simulink model "niof_model"  (R2021a)
settings: Solver=ode23tb  StartTime=0.0  StopTime=2  RelTol=1e-3
values from neighbouring files (symbols this model uses):
  h0 = ds.DateTime(1).Hour + ds.DateTime(1).Minute/60    [compiler_niof_model.m]
  S_area_hole = 0.01    [set_params_blocks.m]
undefined symbols (not defined in the file or in its folder): crop_GH1_NFT_slot1___C, crop_GH1_NFT_slot1___N, crop_GH1_NFT_slot1___R, crop_GH1_NFT_slot2___C, crop_GH1_NFT_slot2___N, crop_GH1_NFT_slot2___R, crop_GH1_NFT_slot3___C, crop_GH1_NFT_slot3___N, crop_GH1_NFT_slot3___R, crop_GH1_NFT_slot4___C, crop_GH1_NFT_slot4___N, crop_GH1_NFT_slot4___R, crop_GH1_RF_slot1___C, crop_GH1_RF_slot1___N, crop_GH1_RF_slot1___R, crop_GH1_RF_slot2___C, crop_GH1_RF_slot2___N, crop_GH1_RF_slot2___R, crop_GH1_RF_slot3___C, crop_GH1_RF_slot3___N, crop_GH1_RF_slot3___R, crop_GH1_RF_slot4___C, crop_GH1_RF_slot4___N, crop_GH1_RF_slot4___R, crop_GH2_RF_slot1___C, crop_GH2_RF_slot1___N, crop_GH2_RF_slot1___R, crop_GH2_RF_slot2___C, crop_GH2_RF_slot2___N, crop_GH2_RF_slot2___R, crop_GH2_RF_slot3___C, crop_GH2_RF_slot3___N, crop_GH2_RF_slot3___R, crop_GH2_RF_slot4___C, crop_GH2_RF_slot4___N, crop_GH2_RF_slot4___R, crop_GH2_TRAD_slot1___C, crop_GH2_TRAD_slot1___N, crop_GH2_TRAD_slot1___R, crop_GH2_TRAD_slot2___C, crop_GH2_TRAD_slot2___N, crop_GH2_TRAD_slot2___R, crop_GH2_TRAD_slot3___C, crop_GH2_TRAD_slot3___N, crop_GH2_TRAD_slot3___R, crop_GH2_TRAD_slot4___C, crop_GH2_TRAD_slot4___N, crop_GH2_TRAD_slot4___R, fish, GH3_Tank1_tend, GH3_Tank2_tend, GH3_Tank3_tend, GH3_Tank4_tend, tp_biofilter___T, tp_fish_C___T, tp_fish_M___T, tp_fish_S___T, tp_fish_T___T, tp_GH1_bio___T, tp_GH1_NFT___T ... (+3)
libraries: HORTISIM x152
(part 1 of 4)
settings Model: Creator=djoroya  LastModifiedBy=djoroya
settings SolverCC: MinimalZcImpactIntegration=on
settings DataIOCC: SaveFormat=StructureWithTime  ReturnWorkspaceOutputsName=tpa3f80949_6031_4c8f_ac4c_761b248f1577
settings DebuggingCC: UnconnectedInputMsg=none  UnconnectedOutputMsg=none  UnconnectedLineMsg=none  UnderSpecifiedDimensionMsg=warning
settings HardwareCC: TargetBitPerLong=64  TargetBitPerPointer=64  TargetBitPerSizeT=64  TargetBitPerPtrDiffT=64  TargetLongLongMode=on  TargetIntDivRoundTo=Zero  TargetEndianess=LittleEndian  TargetWordSize=64  TargetHWDeviceType=MATLAB Host  ProdEqTarget=off
settings RTWCC: Description=Rapid Simulation Target  SystemTargetFile=rsim.tlc  TemplateMakefile=rsim_default_tmf
settings CodeAppCC: GenerateComments=off  SimulinkBlockComments=off
settings RSimTargetCC: TargetLangStandard=C99 (ISO)

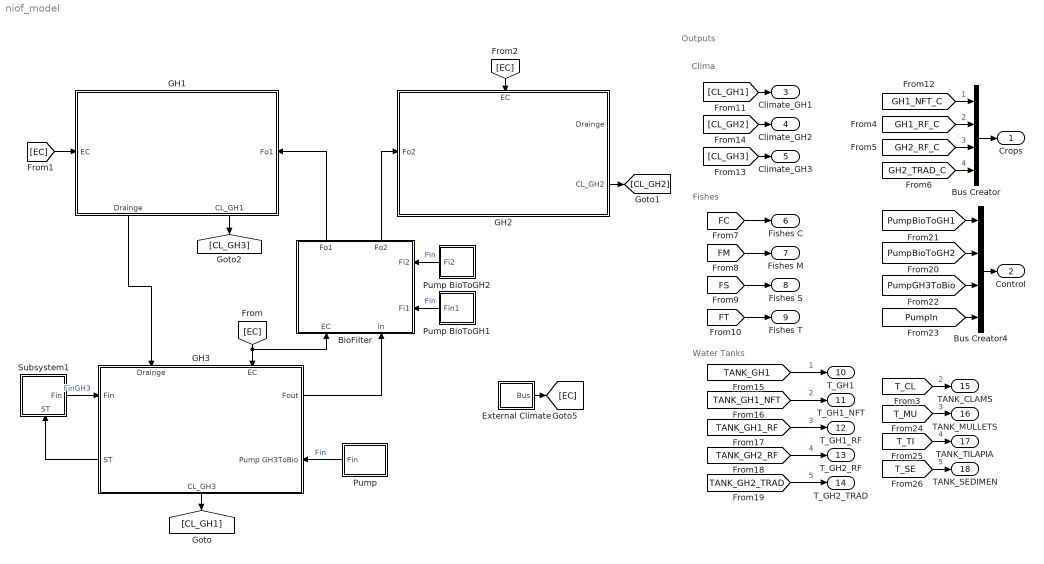
== system niof_model ==
  note: Clima
  note: Water Tanks
  note: Outputs
  note: Fishes
  BioFilter : Subsystem
      settings: PortSchema="{\"entries\":[{\"content\":{\"sides\":[{\"content\":{\"connectorIds\":[]},\"type\":\"ConnectorPlacement.EquallySpacedRectSide\",\"uuid\":\"39de7e6f-241b-402f-a120-18892c124752\"},{\"content\":{\"connectorIds\":[\"In3\",\"In4\"],\"side\":\"RIGHT\"},\"type\":\"ConnectorPlacement.EquallySpacedRectSide\",\"uuid\":\"cefc2988-7ee7-4e24-926e-b8e4989b17f9\"},{\"content\":{\"connectorIds\":[\"Out1\",\"Out2\"],\"side\":\"TOP\"},\"type\":\"ConnectorPlacement.EquallySpacedRectSide\",\"uuid\":\"4036c4c8-5802-453b-98d5-164c4771b92f\"},{\"content\":{\"connectorIds\":[\"In1\",\"In2\"],\"side\":\"BOTTOM\"},\"type\":\"ConnectorPlacement.EquallySpacedRectSide\",\"uuid\":\"379a93f8-bf00-465a-a0f2-a3fe498cb65a\"}]},\"type\":\"ConnectorPlacement.EquallySpacedConnector\",\"uuid\":\"a3e40081-564f-4c6d-9212-7fcf3036ef72\"}],\"packageUris\":[\"http://schema.mathworks.com/mf0/Connector/R2020b\"],\"version\":\"1.0\"}"
  Bus Creator : BusCreator  Inputs=4
  Bus Creator4 : BusCreator  Inputs=4
  External Climate : Subsystem
  GH1 : Subsystem
      settings: PortSchema="{\"entries\":[{\"content\":{\"sides\":[{\"content\":{\"connectorIds\":[\"In1\"]},\"type\":\"ConnectorPlacement.EquallySpacedRectSide\",\"uuid\":\"f96e7fae-faa6-4c45-94ca-623160b74f18\"},{\"content\":{\"connectorIds\":[\"In2\"],\"side\":\"RIGHT\"},\"type\":\"ConnectorPlacement.EquallySpacedRectSide\",\"uuid\":\"cb53bd10-123e-4148-bfa4-80436b7b153d\"},{\"content\":{\"connectorIds\":[],\"side\":\"TOP\"},\"type\":\"ConnectorPlacement.EquallySpacedRectSide\",\"uuid\":\"63bb56bc-b382-4b43-9081-bb2d51c32075\"},{\"content\":{\"connectorIds\":[\"Out1\",\"Out2\"],\"side\":\"BOTTOM\"},\"type\":\"ConnectorPlacement.EquallySpacedRectSide\",\"uuid\":\"67dc5313-4d07-4554-a853-f934e5f830b0\"}]},\"type\":\"ConnectorPlacement.EquallySpacedConnector\",\"uuid\":\"a823a839-de0c-41cf-8d5c-d5714b085e52\"}],\"packageUris\":[\"http://schema.mathworks.com/mf0/Connector/R2020b\"],\"version\":\"1.0\"}"
  GH2 : Subsystem
      settings: PortSchema="{\"entries\":[{\"content\":{\"sides\":[{\"content\":{\"connectorIds\":[\"In1\"]},\"type\":\"ConnectorPlacement.EquallySpacedRectSide\",\"uuid\":\"f96e7fae-faa6-4c45-94ca-623160b74f18\"},{\"content\":{\"connectorIds\":[\"Out1\",\"Out2\"],\"side\":\"RIGHT\"},\"type\":\"ConnectorPlacement.EquallySpacedRectSide\",\"uuid\":\"cb53bd10-123e-4148-bfa4-80436b7b153d\"},{\"content\":{\"connectorIds\":[\"In2\"],\"side\":\"TOP\"},\"type\":\"ConnectorPlacement.EquallySpacedRectSide\",\"uuid\":\"63bb56bc-b382-4b43-9081-bb2d51c32075\"},{\"content\":{\"connectorIds\":[],\"side\":\"BOTTOM\"},\"type\":\"ConnectorPlacement.EquallySpacedRectSide\",\"uuid\":\"67dc5313-4d07-4554-a853-f934e5f830b0\"}]},\"type\":\"ConnectorPlacement.EquallySpacedConnector\",\"uuid\":\"a823a839-de0c-41cf-8d5c-d5714b085e52\"}],\"packageUris\":[\"http://schema.mathworks.com/mf0/Connector/R2020b\"],\"version\":\"1.0\"}"
  GH3 : Subsystem
      settings: PortSchema="{\"entries\":[{\"content\":{\"sides\":[{\"content\":{\"connectorIds\":[\"In1\",\"Out3\"]},\"type\":\"ConnectorPlacement.EquallySpacedRectSide\",\"uuid\":\"81ee264a-41e1-40c0-ab1d-9f5a989c7824\"},{\"content\":{\"connectorIds\":[\"Out1\",\"In4\"],\"side\":\"RIGHT\"},\"type\":\"ConnectorPlacement.EquallySpacedRectSide\",\"uuid\":\"6f93fb8e-2d1c-4265-8b9a-fc3ac97daf53\"},{\"content\":{\"connectorIds\":[\"In2\",\"In3\"],\"side\":\"TOP\"},\"type\":\"ConnectorPlacement.EquallySpacedRectSide\",\"uuid\":\"a3cd6f92-7543-4360-a672-0bbe0cd8561c\"},{\"content\":{\"connectorIds\":[\"Out2\"],\"side\":\"BOTTOM\"},\"type\":\"ConnectorPlacement.EquallySpacedRectSide\",\"uuid\":\"24dd70c2-9a78-443d-9f3d-70d95e180355\"}]},\"type\":\"ConnectorPlacement.EquallySpacedConnector\",\"uuid\":\"c2201d0a-197a-46d7-9039-6a7936abb698\"}],\"packageUris\":[\"http://schema.mathworks.com/mf0/Connector/R2020b\"],\"version\":\"1.0\"}"
  Pump : Subsystem
  Pump BioToGH1 : Subsystem
  Pump BioToGH2 : Subsystem
  Subsystem1 : Subsystem
      settings: PortSchema="{\"entries\":[{\"content\":{\"sides\":[{\"content\":{\"connectorIds\":[]},\"type\":\"ConnectorPlacement.EquallySpacedRectSide\",\"uuid\":\"9a0d525f-008d-4bea-82c7-ff44bdf3c7a1\"},{\"content\":{\"connectorIds\":[\"Out1\"],\"side\":\"RIGHT\"},\"type\":\"ConnectorPlacement.EquallySpacedRectSide\",\"uuid\":\"3b01d65a-c3f3-4d47-b396-44b5c3b80049\"},{\"content\":{\"connectorIds\":[],\"side\":\"TOP\"},\"type\":\"ConnectorPlacement.EquallySpacedRectSide\",\"uuid\":\"5f7d9f63-0ae7-4a14-b423-83c3827e552d\"},{\"content\":{\"connectorIds\":[\"In1\"],\"side\":\"BOTTOM\"},\"type\":\"ConnectorPlacement.EquallySpacedRectSide\",\"uuid\":\"b4e81995-be21-4f86-9bdb-ec727bfc31aa\"}]},\"type\":\"ConnectorPlacement.EquallySpacedConnector\",\"uuid\":\"2d17a637-3468-41a4-99e0-95edda826c96\"}],\"packageUris\":[\"http://schema.mathworks.com/mf0/Connector/R2020b\"],\"version\":\"1.0\"}"
  Crops : Outport  PortDimensions=62*4*4
  Control : Outport  Port=2
  Climate_GH1 : Outport  Port=3
  Climate_GH2 : Outport  Port=4
  Climate_GH3 : Outport  Port=5
  Fishes C : Outport  Port=6
  Fishes M : Outport  Port=7
  Fishes S : Outport  Port=8
  Fishes T : Outport  Port=9
  T_GH1 : Outport  Port=10
  T_GH1_NFT : Outport  Port=11
  T_GH1_RF : Outport  Port=12
  T_GH2_RF : Outport  Port=13
  T_GH2_TRAD : Outport  Port=14
  TANK_CLAMS : Outport  Port=15
  TANK_MULLETS : Outport  Port=16
  TANK_TILAPIA : Outport  Port=17
  TANK_SEDIMEN : Outport  Port=18
  wires:
  Subsystem1/1(Fin) -> GH3/1(Fin)  "FinGH3"
  Pump/1(Fin) -> GH3/4(Pump GH3ToBio)  "Fin"
  External Climate/1(Bus) -> [EC]
  [EC] -> BioFilter/1(EC), GH3/3(EC)
  Pump BioToGH1/1(Fin1) -> BioFilter/4(Fi1)  "Fin"
  Pump BioToGH2/1(Fi2) -> BioFilter/3(Fi2)  "Fin"
  GH3/1(Fout) -> BioFilter/2(in)
  [EC] -> GH1/1(EC)
  [EC] -> GH2/2(EC)
  BioFilter/1(Fo1) -> GH1/2(Fo1)
  BioFilter/2(Fo2) -> GH2/1(Fo2)
  GH1/1(Drainge) -> GH3/2(Drainge)
  GH3/3(ST) -> Subsystem1/1(ST)
  Bus Creator/1 -> Crops/1
  [GH1_NFT_C] -> Bus Creator/1  "1"
  [GH1_RF_C] -> Bus Creator/2  "2"
  [GH2_RF_C] -> Bus Creator/3  "3"
  [GH2_TRAD_C] -> Bus Creator/4  "4"
  [FC] -> Fishes C/1
  [FM] -> Fishes M/1
  [FS] -> Fishes S/1
  [FT] -> Fishes T/1
  [TANK_GH1_NFT] -> T_GH1_NFT/1  "2"
  [TANK_GH1_RF] -> T_GH1_RF/1  "3"
  [TANK_GH2_RF] -> T_GH2_RF/1  "4"
  [TANK_GH2_TRAD] -> T_GH2_TRAD/1  "5"
  [PumpBioToGH1] -> Bus Creator4/1
  [PumpBioToGH2] -> Bus Creator4/2
  [PumpGH3ToBio] -> Bus Creator4/3
  [PumpIn] -> Bus Creator4/4
  Bus Creator4/1 -> Control/1
  [TANK_GH1] -> T_GH1/1  "1"
  GH3/2(CL_GH3) -> [CL_GH1]
  GH2/2(CL_GH2) -> [CL_GH2]
  GH1/2(CL_GH1) -> [CL_GH3]
  [CL_GH1] -> Climate_GH1/1
  [CL_GH2] -> Climate_GH2/1
  [CL_GH3] -> Climate_GH3/1
  [T_CL] -> TANK_CLAMS/1  "2"
  [T_MU] -> TANK_MULLETS/1  "3"
  [T_SE] -> TANK_SEDIMEN/1  "5"
  [T_TI] -> TANK_TILAPIA/1  "4"

== system niof_model/BioFilter ==
  EC : Inport
  in : Inport  Port=2
  Fi2 : Inport  Port=3
  Fi1 : Inport  Port=4
  Bio Filter : Subsystem
  Bus Selector : BusSelector  OutputSignals=Fout
  Parse : Subsystem
  Selector : Selector  InputPortWidth=2  IndexOptions=Index vector (dialog)  Indices=[1]  OutputSizes=1
  Selector1 : Selector  InputPortWidth=2  IndexOptions=Index vector (dialog)  Indices=[2]  OutputSizes=1
  Tank Model Bio : HORTISIM/Aquaculture/Models/Tank Model  S=tp_biofilter___S  h_max=tp_biofilter___h_max  wall_gain=tp_biofilter___wall_gain  ThermalConductivityWall=tp_biofilter___ThermalConductivityWall  Tsubwall=tp_biofilter___Tsubwall  h=tp_biofilter___h  X=tp_biofilter___X  T=tp_biofilter___T  Twall=tp_biofilter___Twall  d_t=tp_biofilter___d_t
      settings: SourceProductName=Horti Simulator
      mask Display: image('water_tank.png'); % Use "Edit Image" on toolstrip to change.
  Vector Concatenate : Concatenate  Mode=Multidimensional array
  Zero Element Flow : HORTISIM/Other  Functions/Zero Element Flow  SystemSampleTime=-1  VariantActivationTime=update diagram  Latency=0  AutoFrameSizeCalculation=off
      settings: SourceProductName=Horti Simulator
  Fo1 : Outport
  Fo2 : Outport  Port=2
  wires:
  Fi2/1 -> Vector Concatenate/2
  in/1 -> Tank Model Bio/1
  Parse/1(Clima) -> Tank Model Bio/3
  Bus Selector/1 -> Selector/1, Selector1/1  "<Fout>"
  Zero Element Flow/1 -> Tank Model Bio/2
  Selector1/1 -> Fo2/1
  Tank Model Bio/1 -> Bus Selector/1  "WT Bio"
  EC/1 -> Parse/1(EC)
  Vector Concatenate/1 -> Tank Model Bio/4
  Fi1/1 -> Vector Concatenate/1
  Selector/1 -> Fo1/1
  Bio Filter/1(Out1) -> Tank Model Bio/5

== system niof_model/External Climate ==
  Constant : Constant  Value=440
  Demux : Demux
  From Workspace : FromWorkspace  VariableName=S01_EC
  Scalar2Bus ExternalClimate : HORTISIM/Other  Functions/Scalar2Bus ExternalClimate  SystemSampleTime=-1  VariantActivationTime=update diagram  Latency=0  AutoFrameSizeCalculation=off
      settings: SourceProductName=Horti Simulator
  Bus : Outport
  wires:
  Scalar2Bus ExternalClimate/1 -> Bus/1
  Demux/3 -> Scalar2Bus ExternalClimate/3
  Demux/1 -> Scalar2Bus ExternalClimate/1
  Demux/2 -> Scalar2Bus ExternalClimate/2
  Constant/1 -> Scalar2Bus ExternalClimate/5
  Demux/4 -> Scalar2Bus ExternalClimate/4
  From Workspace/1 -> Demux/1

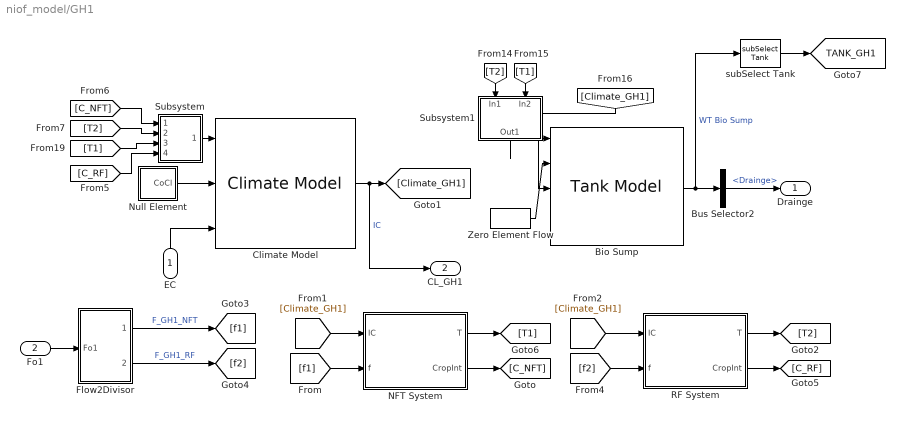
== system niof_model/GH1 ==
  EC : Inport
  Fo1 : Inport  Port=2
  Bio Sump : HORTISIM/Aquaculture/Models/Tank Model  S=tp_GH1_bio___S  h_max=tp_GH1_bio___h_max  wall_gain=tp_GH1_bio___wall_gain  ThermalConductivityWall=tp_GH1_bio___ThermalConductivityWall  Tsubwall=tp_GH1_bio___Tsubwall  h=tp_GH1_bio___h  X=tp_GH1_bio___X  T=tp_GH1_bio___T  Twall=tp_GH1_bio___Twall  d_t=tp_GH1_bio___d_t
      settings: SourceProductName=Horti Simulator
  Bus Selector2 : BusSelector  OutputSignals=Drainge
  Climate Model : HORTISIM/Climate/Models/Climate Model  hour0=climate_GH1___hour0  G0=climate_GH1___G0  T0=climate_GH1___T0  H=climate_GH1___H  A_f=climate_GH1___A_f  A_c=climate_GH1___A_c  minWindows=climate_GH1___minWindows  lam_s=climate_GH1___lam_s  c_s=climate_GH1___c_s  l_s=climate_GH1___l_s  rhod_s=climate_GH1___rhod_s  int_air_speed=climate_GH1___int_air_speed  alpha_i=climate_GH1___alpha_i  alpha_c=climate_GH1___alpha_c  tau_c=climate_GH1___tau_c  alpha_f=climate_GH1___alpha_f  d_c=climate_GH1___d_c  cd_c=climate_GH1___cd_c  T_ss=climate_GH1___T_ss
      settings: SourceProductName=Horti Simulator
  Flow2Divisor : Subsystem
  NFT System : Subsystem
  Null Element : Subsystem
  RF System : Subsystem
  Subsystem : Subsystem
  Subsystem1 : Subsystem
  Zero Element Flow : HORTISIM/Other  Functions/Zero Element Flow  SystemSampleTime=-1  VariantActivationTime=update diagram  Latency=0  AutoFrameSizeCalculation=off
      settings: SourceProductName=Horti Simulator
  subSelect Tank : HORTISIM/Other  Functions/subSelect  Tank  SystemSampleTime=-1  VariantActivationTime=update diagram  Latency=0  AutoFrameSizeCalculation=off
      settings: SourceProductName=Horti Simulator
  Drainge : Outport
  CL_GH1 : Outport  Port=2
  tag scope: TANK_GH1=global
  wires:
  Fo1/1 -> Flow2Divisor/1(Fo1)
  Flow2Divisor/1(Out1) -> [f1]  "F_GH1_NFT"
  Flow2Divisor/2(Out2) -> [f2]  "F_GH1_RF"
  [f2] -> RF System/2(f)
  [Climate_GH1] -> RF System/1(IC)
  RF System/1(T) -> [T2]
  [f1] -> NFT System/2(f)
  [Climate_GH1] -> NFT System/1(IC)
  NFT System/1(T) -> [T1]
  RF System/2(CropInt) -> [C_RF]
  NFT System/2(CropInt) -> [C_NFT]
  Null Element/1(CoCl) -> Climate Model/2
  Climate Model/1 -> CL_GH1/1, [Climate_GH1]  "IC"
  EC/1 -> Climate Model/3
  [C_NFT] -> Subsystem/1(In1)
  [T2] -> Subsystem/2(In2)
  [T1] -> Subsystem/3(In3)
  [C_RF] -> Subsystem/4(In4)
  Subsystem/1(CoCl) -> Climate Model/1
  Zero Element Flow/1 -> Bio Sump/2
  Bus Selector2/1 -> Drainge/1  "<Drainge>"
  Bio Sump/1 -> subSelect Tank/1, Bus Selector2/1  "WT Bio Sump"
  [Climate_GH1] -> Bio Sump/3
  [T2] -> Subsystem1/1(In1)
  [T1] -> Subsystem1/2(In2)
  Subsystem1/1(Out1) -> Bio Sump/1
  subSelect Tank/1 -> [TANK_GH1]

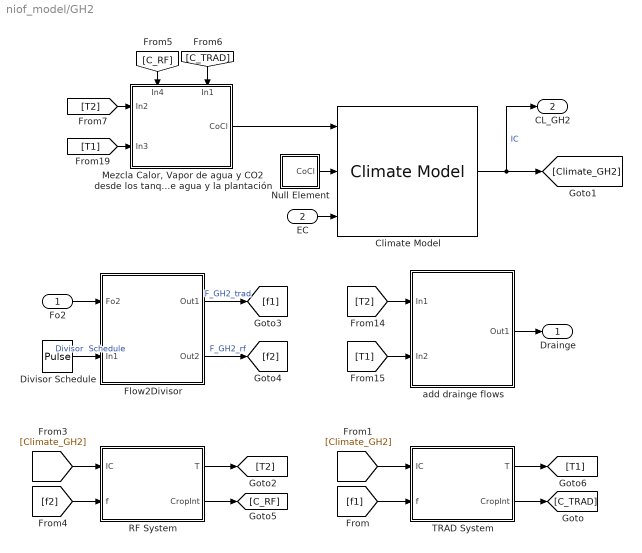
== system niof_model/GH2 ==
  Fo2 : Inport
  EC : Inport  Port=2
  Climate Model : HORTISIM/Climate/Models/Climate Model  hour0=climate_GH2___hour0  G0=climate_GH2___G0  T0=climate_GH2___T0  H=climate_GH2___H  A_f=climate_GH2___A_f  A_c=climate_GH2___A_c  minWindows=climate_GH2___minWindows  lam_s=climate_GH2___lam_s  c_s=climate_GH2___c_s  l_s=climate_GH2___l_s  rhod_s=climate_GH2___rhod_s  int_air_speed=climate_GH2___int_air_speed  alpha_i=climate_GH2___alpha_i  alpha_c=climate_GH2___alpha_c  tau_c=climate_GH2___tau_c  alpha_f=climate_GH2___alpha_f  d_c=climate_GH2___d_c  cd_c=climate_GH2___cd_c  T_ss=climate_GH2___T_ss
      settings: SourceProductName=Horti Simulator
  Divisor Schedule : DiscretePulseGenerator  PulseType=Time based  Period=7  PulseWidth=100/7  PhaseDelay=8/24-h0
  Flow2Divisor : Subsystem
  "Mezcla Calor, Vapor de agua y CO2 desde los tanques de agua y la plantación" : Subsystem
      settings: PortSchema="{\"entries\":[{\"content\":{\"sides\":[{\"content\":{\"connectorIds\":[\"In1\",\"In2\"]},\"type\":\"ConnectorPlacement.EquallySpacedRectSide\",\"uuid\":\"19434035-201c-4d1e-b085-add0f5d76683\"},{\"content\":{\"connectorIds\":[\"Out1\"],\"side\":\"RIGHT\"},\"type\":\"ConnectorPlacement.EquallySpacedRectSide\",\"uuid\":\"bba1eca2-c9f3-4d99-84f3-6a563e445b18\"},{\"content\":{\"connectorIds\":[\"In3\",\"In4\"],\"side\":\"TOP\"},\"type\":\"ConnectorPlacement.EquallySpacedRectSide\",\"uuid\":\"0c3973cd-a057-4788-9737-1d39699ad24a\"}]},\"type\":\"ConnectorPlacement.EquallySpacedConnector\",\"uuid\":\"7a49bd96-3016-4969-a817-6dbc9b87987e\"}],\"packageUris\":[\"http://schema.mathworks.com/mf0/Connector/R2020b\"],\"version\":\"1.0\"}"
  Null Element : Subsystem
  RF System : Subsystem
  TRAD System : Subsystem
  add drainge flows : Subsystem
  Drainge : Outport
  CL_GH2 : Outport  Port=2
  wires:
  Fo2/1 -> Flow2Divisor/1(Fo2)
  Flow2Divisor/1(Out1) -> [f1]  "F_GH2_trad"
  Flow2Divisor/2(Out2) -> [f2]  "F_GH2_rf"
  Divisor Schedule/1 -> Flow2Divisor/2(In1)  "Divisor  Schedule"
  [f2] -> RF System/2(f)
  [Climate_GH2] -> TRAD System/1(IC)
  RF System/1(T) -> [T2]
  [Climate_GH2] -> RF System/1(IC)
  RF System/2(CropInt) -> [C_RF]
  TRAD System/2(CropInt) -> [C_TRAD]
  TRAD System/1(T) -> [T1]
  [f1] -> TRAD System/2(f)
  Null Element/1(CoCl) -> Climate Model/2
  Climate Model/1 -> CL_GH2/1, [Climate_GH2]  "IC"
  EC/1 -> Climate Model/3
  [C_TRAD] -> "Mezcla Calor, Vapor de agua y CO2 desde los tanques de agua y la plantación"/4(In1)
  [T2] -> "Mezcla Calor, Vapor de agua y CO2 desde los tanques de agua y la plantación"/1(In2)
  [T1] -> "Mezcla Calor, Vapor de agua y CO2 desde los tanques de agua y la plantación"/2(In3)
  [C_RF] -> "Mezcla Calor, Vapor de agua y CO2 desde los tanques de agua y la plantación"/3(In4)
  "Mezcla Calor, Vapor de agua y CO2 desde los tanques de agua y la plantación"/1(CoCl) -> Climate Model/1
  [T2] -> add drainge flows/1(In1)
  [T1] -> add drainge flows/2(In2)
  add drainge flows/1(Out1) -> Drainge/1

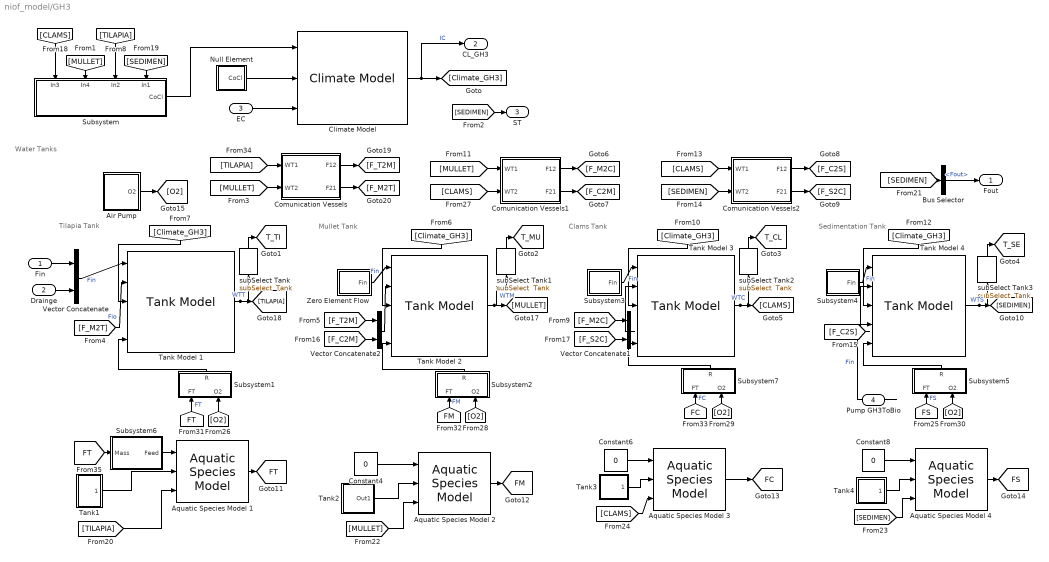
== system niof_model/GH3 ==
  note: Water Tanks
  note: Tilapia Tank
  note: Clams Tank
  note: Mullet Tank
  note: Sedimentation Tank
  Fin : Inport
  Drainge : Inport  Port=2
  EC : Inport  Port=3
  Pump GH3ToBio : Inport  Port=4
  Air Pump : Subsystem
  Aquatic Species Model 1 : HORTISIM/Aquaculture/Models/Aquatic Species Model  rfish=ratio.tilapia  mfishsat=mass_sat.tilapia  a_max=GH3_Tank1_tend + 1  a0=0  m0=fish.tilapia.Mass(1)  A_R=1e-3*[1 0 0 0 0 0 -1 1]'  B_R=1e-3*[1 0 0 0 0 0 -1 1]'
      settings: SourceProductName=Horti Simulator
  Aquatic Species Model 2 : HORTISIM/Aquaculture/Models/Aquatic Species Model  rfish=ratio.mullet  mfishsat=mass_sat.mullet  a_max=GH3_Tank2_tend + 1  a0=0  m0=fish.mullet.Mass(1)  A_R=1e-3*[1 0 0 0 0 0 -1 1]'  B_R=1e-3*[1 0 0 0 0 0 -1 1]'
      settings: SourceProductName=Horti Simulator
  Aquatic Species Model 3 : HORTISIM/Aquaculture/Models/Aquatic Species Model  rfish=ratio.clams  mfishsat=mass_sat.clams  a_max=GH3_Tank3_tend + 1  a0=0  m0=fish.clams.Mass(1)  A_R=1e-3*[1 0 0 0 0 0 -1 1]'  B_R=1e-3*[1 0 0 0 0 0 -1 1]'
      settings: SourceProductName=Horti Simulator
  Aquatic Species Model 4 : HORTISIM/Aquaculture/Models/Aquatic Species Model  rfish=ratio.silver  mfishsat=mass_sat.silver  a_max=GH3_Tank4_tend + 1  a0=0  m0=fish.silver.Mass(1)  A_R=1e-3*[1 0 0 0 0 0 -1 1]'  B_R=1e-3*[1 0 0 0 0 0 -1 1]'
      settings: SourceProductName=Horti Simulator
  Bus Selector : BusSelector  OutputSignals=Fout
  Climate Model : HORTISIM/Climate/Models/Climate Model  hour0=climate_GH3___hour0  G0=climate_GH3___G0  T0=climate_GH3___T0  H=climate_GH3___H  A_f=climate_GH3___A_f  A_c=climate_GH3___A_c  minWindows=climate_GH3___minWindows  lam_s=climate_GH3___lam_s  c_s=climate_GH3___c_s  l_s=climate_GH3___l_s  rhod_s=climate_GH3___rhod_s  int_air_speed=climate_GH3___int_air_speed  alpha_i=climate_GH3___alpha_i  alpha_c=climate_GH3___alpha_c  tau_c=climate_GH3___tau_c  alpha_f=climate_GH3___alpha_f  d_c=climate_GH3___d_c  cd_c=climate_GH3___cd_c  T_ss=climate_GH3___T_ss
      settings: SourceProductName=Horti Simulator
  Comunication Vessels : Subsystem  mask{S=S_area_hole}
  Comunication Vessels1 : Subsystem  mask{S=S_area_hole}
  Comunication Vessels2 : Subsystem  mask{S=S_area_hole}
  Constant4 : Constant  Value=0
  Constant6 : Constant  Value=0
  Constant8 : Constant  Value=0
  Null Element : Subsystem
  Subsystem : Subsystem
      settings: PortSchema="{\"entries\":[{\"content\":{\"sides\":[{\"content\":{\"connectorIds\":[]},\"type\":\"ConnectorPlacement.EquallySpacedRectSide\",\"uuid\":\"d0110122-4c0e-4050-9905-351100dfb2f8\"},{\"content\":{\"connectorIds\":[\"Out1\"],\"side\":\"RIGHT\"},\"type\":\"ConnectorPlacement.EquallySpacedRectSide\",\"uuid\":\"5eb4c138-aba2-4968-a926-5140e929ef74\"},{\"content\":{\"connectorIds\":[\"In1\",\"In2\",\"In3\",\"In4\"],\"side\":\"TOP\"},\"type\":\"ConnectorPlacement.EquallySpacedRectSide\",\"uuid\":\"102db217-6442-4bf3-9377-05d6ceeffd2a\"}]},\"type\":\"ConnectorPlacement.EquallySpacedConnector\",\"uuid\":\"fec43415-4143-4543-8db6-6efa996130a9\"}],\"packageUris\":[\"http://schema.mathworks.com/mf0/Connector/R2020b\"],\"version\":\"1.0\"}"
  Subsystem1 : Subsystem
  Subsystem2 : Subsystem
  Subsystem3 : Subsystem
  Subsystem4 : Subsystem
  Subsystem5 : Subsystem
  Subsystem6 : Subsystem  mask{FCR=1e-4}
  Subsystem7 : Subsystem
  Tank Model 1 : HORTISIM/Aquaculture/Models/Tank Model  S=tp_fish_T___S  h_max=tp_fish_T___h_max  wall_gain=tp_fish_T___wall_gain  ThermalConductivityWall=tp_fish_T___ThermalConductivityWall  Tsubwall=tp_fish_T___Tsubwall  h=tp_fish_T___h  X=tp_fish_T___X  T=tp_fish_T___T  Twall=tp_fish_T___Twall  d_t=tp_fish_T___d_t
      settings: SourceProductName=Horti Simulator
  Tank Model 2 : HORTISIM/Aquaculture/Models/Tank Model  S=tp_fish_M___S  h_max=tp_fish_M___h_max  wall_gain=tp_fish_M___wall_gain  ThermalConductivityWall=tp_fish_M___ThermalConductivityWall  Tsubwall=tp_fish_M___Tsubwall  h=tp_fish_M___h  X=tp_fish_M___X  T=tp_fish_M___T  Twall=tp_fish_M___Twall  d_t=tp_fish_M___d_t
      settings: SourceProductName=Horti Simulator
      mask Display: image('water_tank.png'); % Use "Edit Image" on toolstrip to change.
  Tank Model 3 : HORTISIM/Aquaculture/Models/Tank Model  S=tp_fish_C___S  h_max=tp_fish_C___h_max  wall_gain=tp_fish_C___wall_gain  ThermalConductivityWall=tp_fish_C___ThermalConductivityWall  Tsubwall=tp_fish_C___Tsubwall  h=tp_fish_C___h  X=tp_fish_C___X  T=tp_fish_C___T  Twall=tp_fish_C___Twall  d_t=tp_fish_C___d_t
      settings: SourceProductName=Horti Simulator
      mask Display: image('water_tank.png'); % Use "Edit Image" on toolstrip to change.
  Tank Model 4 : HORTISIM/Aquaculture/Models/Tank Model  S=tp_fish_S___S  h_max=tp_fish_S___h_max  wall_gain=tp_fish_S___wall_gain  ThermalConductivityWall=tp_fish_S___ThermalConductivityWall  Tsubwall=tp_fish_S___Tsubwall  h=tp_fish_S___h  X=tp_fish_S___X  T=tp_fish_S___T  Twall=tp_fish_S___Twall  d_t=tp_fish_S___d_t
      settings: SourceProductName=Horti Simulator
      mask Display: image('water_tank.png'); % Use "Edit Image" on toolstrip to change.
  Tank1 : Subsystem
  Tank2 : Subsystem
  Tank3 : Subsystem
  Tank4 : Subsystem
  Vector Concatenate : Concatenate  Mode=Multidimensional array
  Vector Concatenate1 : Concatenate
  Vector Concatenate2 : Concatenate
  Zero Element Flow : Subsystem
  subSelect Tank{,1..3} (4 alike) : HORTISIM/Other  Functions/subSelect  Tank  SystemSampleTime=-1  VariantActivationTime=update diagram  Latency=0  AutoFrameSizeCalculation=off
      settings: SourceProductName=Horti Simulator
  Fout : Outport
  CL_GH3 : Outport  Port=2
  ST : Outport  Port=3
  tag scope: FC=global, FM=global, FS=global, FT=global, T_CL=global, T_MU=global, T_SE=global, T_TI=global
  wires:
  EC/1 -> Climate Model/3
  [SEDIMEN] -> Subsystem/4(In1)
  Climate Model/1 -> CL_GH3/1, [Climate_GH3]  "IC"
  Subsystem/1(CoCl) -> Climate Model/1
  [CLAMS] -> Subsystem/1(In3)
  [MULLET] -> Subsystem/2(In4)
  [TILAPIA] -> Subsystem/3(In2)
  Null Element/1(CoCl) -> Climate Model/2
  Fin/1 -> Vector Concatenate/1
  Drainge/1 -> Vector Concatenate/2
  [SEDIMEN] -> ST/1
  Bus Selector/1 -> Fout/1  "<Fout>"
  Subsystem5/1(R) -> Tank Model 4/5
  [FS] -> Subsystem5/1(FT)  "FS"
  [O2] -> Subsystem5/2(O2)
  Subsystem7/1(R) -> Tank Model 3/5
  [FC] -> Subsystem7/1(FT)  "FC"
  [O2] -> Subsystem7/2(O2)
  Subsystem2/1(R) -> Tank Model 2/5
  [O2] -> Subsystem2/2(O2)
  [FM] -> Subsystem2/1(FT)  "FM"
  Subsystem1/1(R) -> Tank Model 1/5
  [O2] -> Subsystem1/2(O2)
  [FT] -> Subsystem1/1(FT)  "FT"
  Air Pump/1(O2) -> [O2]
  Aquatic Species Model 4/1 -> [FS]
  Aquatic Species Model 3/1 -> [FC]
  Aquatic Species Model 2/1 -> [FM]
  Aquatic Species Model 1/1 -> [FT]
  [FT] -> Subsystem6/1(Mass)
  Subsystem6/1(Feed) -> Aquatic Species Model 1/1
  [MULLET] -> Comunication Vessels/2(WT2)
  [MULLET] -> Comunication Vessels1/1(WT1)
  [CLAMS] -> Comunication Vessels2/1(WT1)
  [Climate_GH3] -> Tank Model 4/3
  [F_C2S] -> Tank Model 4/2
  Comunication Vessels/1(F12) -> [F_T2M]
  [Climate_GH3] -> Tank Model 3/3
  Constant4/1 -> Aquatic Species Model 2/1
  [TILAPIA] -> Comunication Vessels/1(WT1)
  Comunication Vessels2/2(F21) -> [F_S2C]
  [F_M2T] -> Tank Model 1/2  "Fio"
  Vector Concatenate/1 -> Tank Model 1/1  "Fin"
  Vector Concatenate1/1 -> Tank Model 3/2
  Pump GH3ToBio/1 -> Tank Model 4/4  "Fin"
  Tank Model 4/1 -> subSelect Tank3/1, [SEDIMEN]  "WTS"
  Comunication Vessels/2(F21) -> [F_M2T]
  [F_C2M] -> Vector Concatenate2/2
  [CLAMS] -> Comunication Vessels1/2(WT2)
  Subsystem4/1(Fin) -> Tank Model 4/1  "Fin"
  Tank Model 1/1 -> subSelect Tank/1, [TILAPIA]  "WTT"
  Tank Model 2/1 -> subSelect Tank1/1, [MULLET]  "WTM"
  Tank Model 3/1 -> subSelect Tank2/1, [CLAMS]  "WTC"
  Constant8/1 -> Aquatic Species Model 4/1
  [F_T2M] -> Vector Concatenate2/1
  [SEDIMEN] -> Aquatic Species Model 4/3
  [F_M2C] -> Vector Concatenate1/1
  Comunication Vessels1/1(F12) -> [F_M2C]
  Comunication Vessels2/1(F12) -> [F_C2S]
  Constant6/1 -> Aquatic Species Model 3/1
  Zero Element Flow/1(Fin) -> Tank Model 2/1  "Fin"
  [Climate_GH3] -> Tank Model 1/3
  Comunication Vessels1/2(F21) -> [F_C2M]
  Subsystem3/1(Fin) -> Tank Model 3/1  "Fin"
  Vector Concatenate2/1 -> Tank Model 2/2
  [TILAPIA] -> Aquatic Species Model 1/3
  [Climate_GH3] -> Tank Model 2/3
  [F_S2C] -> Vector Concatenate1/2
  [SEDIMEN] -> Comunication Vessels2/2(WT2)
  [CLAMS] -> Aquatic Species Model 3/3
  [SEDIMEN] -> Bus Selector/1
  [MULLET] -> Aquatic Species Model 2/3
  subSelect Tank/1 -> [T_TI]
  subSelect Tank1/1 -> [T_MU]
  subSelect Tank2/1 -> [T_CL]
  subSelect Tank3/1 -> [T_SE]
  Tank1/1(Out1) -> Aquatic Species Model 1/2
  Tank2/1(Out1) -> Aquatic Species Model 2/2
  Tank3/1(Out1) -> Aquatic Species Model 3/2
  Tank4/1(Out1) -> Aquatic Species Model 4/2

== system niof_model/Pump ==
  1h/3600s : Gain  Gain=1/3600
  m3/h : Constant  Value=13
  Fin : Outport
  tag scope: PumpGH3ToBio=global
  wires:
  1h/3600s/1 -> [PumpGH3ToBio], Fin/1  "PumpGH3ToBio"
  m3/h/1 -> 1h/3600s/1

== system niof_model/Pump BioToGH1 ==
  1h/3600s : Gain  Gain=1/3600
  m3/h : Constant  Value=13
  Fin1 : Outport
  tag scope: PumpBioToGH1=global
  wires:
  m3/h/1 -> 1h/3600s/1
  1h/3600s/1 -> [PumpBioToGH1], Fin1/1  "PumpBioToGH1"

== system niof_model/Pump BioToGH2 ==
  1h/3600s : Gain  Gain=1/3600
  Product : Product
  Pulse Generator : DiscretePulseGenerator  PulseType=Time based  Period=1  PulseWidth=7/24*100  PhaseDelay=8/24-h0
  Scope : Scope
  m3/h : Constant  Value=0.1
  Fi2 : Outport
  tag scope: PumpBioToGH2=global
  wires:
  m3/h/1 -> 1h/3600s/1
  Pulse Generator/1 -> Scope/1, Product/1
  1h/3600s/1 -> Product/2  "f"
  Product/1 -> [PumpBioToGH2], Fi2/1  "PumpBioToGH2"

== system niof_model/Subsystem1 ==
  note: m3/s
  note: Well Water1
  ST : Inport
  1h/3600s : Gain  Gain=1/3600
  Abs : Abs  ZeroCross=off
  Bus Creator1 : BusCreator  Inputs=3  OutDataTypeStr=Bus: FLOW  NonVirtualBus=on
  Bus Selector : BusSelector  OutputSignals=h
  Constant : Constant  Value=0.8
  Minus : Sum  Inputs=+-
  Product : Product
  Product1 : Product
  Pulse Generator : DiscretePulseGenerator  PulseType=Time based  Period=1  PulseWidth=3/(24)*100  PhaseDelay=8/24-h0
  Scope : Scope
  "[Kelvin]1" : Constant  Value=273.15 + 20
  kg/m^3 : Constant  Value=0.1 + zeros(8,1)
  m3/h : Constant  Value=100
  m3/h1 : Constant  Value=18
  Fin : Outport
  tag scope: PumpIn=global
  wires:
  Bus Creator1/1 -> Fin/1
  kg/m^3/1 -> Bus Creator1/3  "X"
  "[Kelvin]1"/1 -> Bus Creator1/2  "T"
  Product/1 -> [PumpIn], Bus Creator1/1  "f"
  1h/3600s/1 -> Product/2
  Pulse Generator/1 -> Scope/1, Product/1
  ST/1 -> Bus Selector/1
  Bus Selector/1 -> Minus/2  "<h>"
  Constant/1 -> Minus/1
  Product1/1 -> 1h/3600s/1
  m3/h/1 -> Product1/1
  Minus/1 -> Abs/1
  Abs/1 -> Product1/2

== system niof_model/BioFilter/Bio Filter ==
  note: %N K Ca Mg P S O2 TSS
  Constant : Constant  Value=[0 0 0 0 0 0 1 0]'  VectorParams1D=off
  Gain : Gain
  Out1 : Outport
  wires:
  Constant/1 -> Gain/1
  Gain/1 -> Out1/1

== system niof_model/BioFilter/Parse ==
  EC : Inport
  Bus Selector : BusSelector  OutputSignals=Temp,HR,Wind
  Gain : Gain  Gain=1/100
  Product : Product
  Temp2SatDensity : HORTISIM/Other  Functions/Temp2SatDensity  SystemSampleTime=-1  VariantActivationTime=update diagram  Latency=0  AutoFrameSizeCalculation=off
      settings: SourceProductName=Horti Simulator
  Out Bus Element : Outport  PortName=Clima  Element=Temp.Tair
  Out Bus Element1 : Outport  PortName=Clima  Element=Gas.air_speed
  Out Bus Element2 : Outport  PortName=Clima  Element=Gas.C_w
  wires:
  EC/1 -> Bus Selector/1
  Bus Selector/1 -> Out Bus Element/1, Temp2SatDensity/1  "<Temp>"
  Bus Selector/2 -> Gain/1  "<HR>"
  Temp2SatDensity/1 -> Product/1
  Gain/1 -> Product/2
  Product/1 -> Out Bus Element2/1
  Bus Selector/3 -> Out Bus Element1/1  "<Wind>"

== system niof_model/GH1/Flow2Divisor ==
  Fo1 : Inport
  Bus Creator : BusCreator  Inputs=3  OutDataTypeStr=Bus: FLOW  NonVirtualBus=on
  Bus Creator1 : BusCreator  Inputs=3  OutDataTypeStr=Bus: FLOW  NonVirtualBus=on
  Bus Selector : BusSelector  OutputSignals=f,T,X
  Gain : Gain  Gain=1/2
  Out1 : Outport
  Out2 : Outport  Port=2
  wires:
  Fo1/1 -> Bus Selector/1
  Bus Selector/1 -> Gain/1  "<f>"
  Gain/1 -> [f]
  Bus Selector/2 -> [T]  "<T>"
  Bus Selector/3 -> [X]  "<X>"
  [f] -> Bus Creator/1  "f"
  [T] -> Bus Creator/2  "T"
  Bus Creator/1 -> Out1/1
  [X] -> Bus Creator/3  "X"
  [f] -> Bus Creator1/1  "f"
  [T] -> Bus Creator1/2  "T"
  Bus Creator1/1 -> Out2/1
  [X] -> Bus Creator1/3  "X"

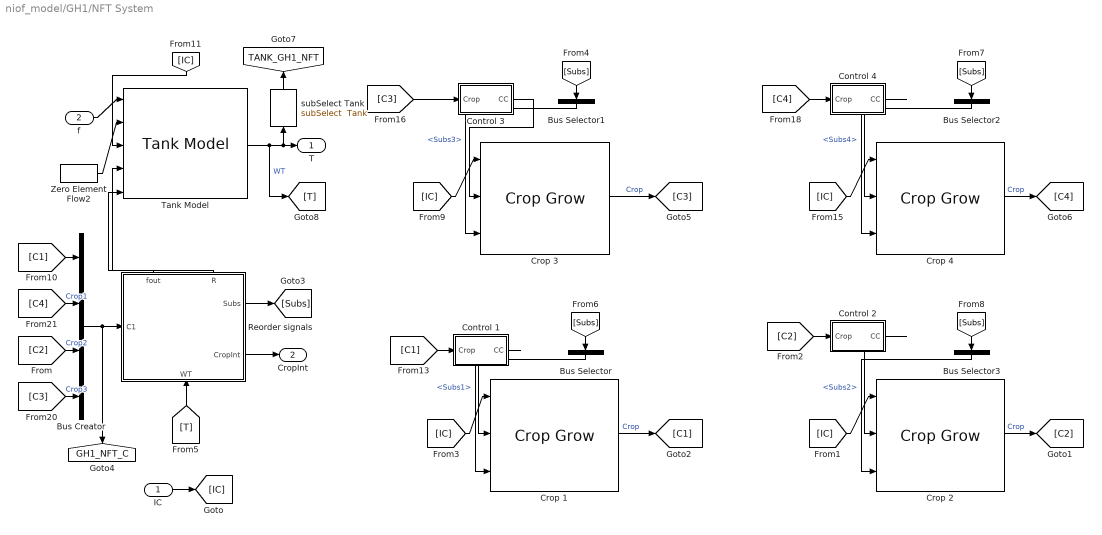
== system niof_model/GH1/NFT System ==
  IC : Inport
  f : Inport  Port=2
  Bus Selector : BusSelector  OutputSignals=Subs1
  Bus Selector1 : BusSelector  OutputSignals=Subs3
  Bus Selector2 : BusSelector  OutputSignals=Subs4
  Bus Selector3 : BusSelector  OutputSignals=Subs2
  Bus Creator : BusCreator  Inputs=4
  Control 1 : Subsystem
  Control 2 : Subsystem
  Control 3 : Subsystem
  Control 4 : Subsystem
  Crop 1 : HORTISIM/Horticulture/Models/Crop Grow  Chi_nutrients=crop_GH1_NFT_slot1___Chi_nutrients  A_v=crop_GH1_NFT_slot1___A_v  plants_density=crop_GH1_NFT_slot1___plants_density  fraction_DM=crop_GH1_NFT_slot1___fraction_DM  min_water_capacity=crop_GH1_NFT_slot1___min_water_capacity  C_buf_max=crop_GH1_NFT_slot1___C_buf_max  T_v_start_fruit=crop_GH1_NFT_slot1___T_v_start_fruit  int_air_speed=crop_GH1_NFT_slot1___int_air_speed  b_N_uptake=crop_GH1_NFT_slot1___b_N_uptake  Tv=crop_GH1_NFT_slot1___Tv  C=crop_GH1_NFT_slot1___C  R=crop_GH1_NFT_slot1___R  Tsum=crop_GH1_NFT_slot1___Tsum  C_wv=crop_GH1_NFT_slot1___C_wv  N=crop_GH1_NFT_slot1___N  rg_fruit=crop_GH1_NFT_slot1___rg_fruit  c_fruit_m=crop_GH1_NFT_slot1___c_fruit_m  c_fruit_g=crop_GH1_NFT_slot1___c_fruit_g  rg_leaf=crop_GH1_NFT_slot1___rg_leaf  c_leaf_m=crop_GH1_NFT_slot1___c_leaf_m  c_leaf_g=crop_GH1_NFT_slot1___c_leaf_g  rg_stem=crop_GH1_NFT_slot1___rg_stem  c_stem_m=crop_GH1_NFT_slot1___c_stem_m  c_stem_g=crop_GH1_NFT_slot1___c_stem_g  VelocityAbsortion=crop_GH1_NFT_slot1___VelocityAbsortion  T_max_v=crop_GH1_NFT_slot1___T_max_v  s_max_T=crop_GH1_NFT_slot1___s_max_T  s_min_T=crop_GH1_NFT_slot1___s_min_T  s_buforg_buf=crop_GH1_NFT_slot1___s_buforg_buf  T_sum_end=crop_GH1_NFT_slot1___T_sum_end  T_max_v24=crop_GH1_NFT_slot1___T_max_v24  T_min_v24=crop_GH1_NFT_slot1___T_min_v24  s_min_T24=crop_GH1_NFT_slot1___s_min_T24  s_max_T24=crop_GH1_NFT_slot1___s_max_T24  T_min_v=crop_GH1_NFT_slot1___T_min_v
      settings: SourceProductName=Horti Simulator
  Crop 2 : HORTISIM/Horticulture/Models/Crop Grow  Chi_nutrients=crop_GH1_NFT_slot2___Chi_nutrients  A_v=crop_GH1_NFT_slot2___A_v  plants_density=crop_GH1_NFT_slot2___plants_density  fraction_DM=crop_GH1_NFT_slot2___fraction_DM  min_water_capacity=crop_GH1_NFT_slot2___min_water_capacity  C_buf_max=crop_GH1_NFT_slot2___C_buf_max  T_v_start_fruit=crop_GH1_NFT_slot2___T_v_start_fruit  int_air_speed=crop_GH1_NFT_slot2___int_air_speed  b_N_uptake=crop_GH1_NFT_slot2___b_N_uptake  Tv=crop_GH1_NFT_slot2___Tv  C=crop_GH1_NFT_slot2___C  R=crop_GH1_NFT_slot2___R  Tsum=crop_GH1_NFT_slot2___Tsum  C_wv=crop_GH1_NFT_slot2___C_wv  N=crop_GH1_NFT_slot2___N  rg_fruit=crop_GH1_NFT_slot2___rg_fruit  c_fruit_m=crop_GH1_NFT_slot2___c_fruit_m  c_fruit_g=crop_GH1_NFT_slot2___c_fruit_g  rg_leaf=crop_GH1_NFT_slot2___rg_leaf  c_leaf_m=crop_GH1_NFT_slot2___c_leaf_m  c_leaf_g=crop_GH1_NFT_slot2___c_leaf_g  rg_stem=crop_GH1_NFT_slot2___rg_stem  c_stem_m=crop_GH1_NFT_slot2___c_stem_m  c_stem_g=crop_GH1_NFT_slot2___c_stem_g  VelocityAbsortion=crop_GH1_NFT_slot2___VelocityAbsortion  T_max_v=crop_GH1_NFT_slot2___T_max_v  s_max_T=crop_GH1_NFT_slot2___s_max_T  s_min_T=crop_GH1_NFT_slot2___s_min_T  s_buforg_buf=crop_GH1_NFT_slot2___s_buforg_buf  T_sum_end=crop_GH1_NFT_slot2___T_sum_end  T_max_v24=crop_GH1_NFT_slot2___T_max_v24  T_min_v24=crop_GH1_NFT_slot2___T_min_v24  s_min_T24=crop_GH1_NFT_slot2___s_min_T24  s_max_T24=crop_GH1_NFT_slot2___s_max_T24  T_min_v=crop_GH1_NFT_slot2___T_min_v
      settings: SourceProductName=Horti Simulator
  Crop 3 : HORTISIM/Horticulture/Models/Crop Grow  Chi_nutrients=crop_GH1_NFT_slot3___Chi_nutrients  A_v=crop_GH1_NFT_slot3___A_v  plants_density=crop_GH1_NFT_slot3___plants_density  fraction_DM=crop_GH1_NFT_slot3___fraction_DM  min_water_capacity=crop_GH1_NFT_slot3___min_water_capacity  C_buf_max=crop_GH1_NFT_slot3___C_buf_max  T_v_start_fruit=crop_GH1_NFT_slot3___T_v_start_fruit  int_air_speed=crop_GH1_NFT_slot3___int_air_speed  b_N_uptake=crop_GH1_NFT_slot3___b_N_uptake  Tv=crop_GH1_NFT_slot3___Tv  C=crop_GH1_NFT_slot3___C  R=crop_GH1_NFT_slot3___R  Tsum=crop_GH1_NFT_slot3___Tsum  C_wv=crop_GH1_NFT_slot3___C_wv  N=crop_GH1_NFT_slot3___N  rg_fruit=crop_GH1_NFT_slot3___rg_fruit  c_fruit_m=crop_GH1_NFT_slot3___c_fruit_m  c_fruit_g=crop_GH1_NFT_slot3___c_fruit_g  rg_leaf=crop_GH1_NFT_slot3___rg_leaf  c_leaf_m=crop_GH1_NFT_slot3___c_leaf_m  c_leaf_g=crop_GH1_NFT_slot3___c_leaf_g  rg_stem=crop_GH1_NFT_slot3___rg_stem  c_stem_m=crop_GH1_NFT_slot3___c_stem_m  c_stem_g=crop_GH1_NFT_slot3___c_stem_g  VelocityAbsortion=crop_GH1_NFT_slot3___VelocityAbsortion  T_max_v=crop_GH1_NFT_slot3___T_max_v  s_max_T=crop_GH1_NFT_slot3___s_max_T  s_min_T=crop_GH1_NFT_slot3___s_min_T  s_buforg_buf=crop_GH1_NFT_slot3___s_buforg_buf  T_sum_end=crop_GH1_NFT_slot3___T_sum_end  T_max_v24=crop_GH1_NFT_slot3___T_max_v24  T_min_v24=crop_GH1_NFT_slot3___T_min_v24  s_min_T24=crop_GH1_NFT_slot3___s_min_T24  s_max_T24=crop_GH1_NFT_slot3___s_max_T24  T_min_v=crop_GH1_NFT_slot3___T_min_v
      settings: SourceProductName=Horti Simulator
  Crop 4 : HORTISIM/Horticulture/Models/Crop Grow  Chi_nutrients=crop_GH1_NFT_slot4___Chi_nutrients  A_v=crop_GH1_NFT_slot4___A_v  plants_density=crop_GH1_NFT_slot4___plants_density  fraction_DM=crop_GH1_NFT_slot4___fraction_DM  min_water_capacity=crop_GH1_NFT_slot4___min_water_capacity  C_buf_max=crop_GH1_NFT_slot4___C_buf_max  T_v_start_fruit=crop_GH1_NFT_slot4___T_v_start_fruit  int_air_speed=crop_GH1_NFT_slot4___int_air_speed  b_N_uptake=crop_GH1_NFT_slot4___b_N_uptake  Tv=crop_GH1_NFT_slot4___Tv  C=crop_GH1_NFT_slot4___C  R=crop_GH1_NFT_slot4___R  Tsum=crop_GH1_NFT_slot4___Tsum  C_wv=crop_GH1_NFT_slot4___C_wv  N=crop_GH1_NFT_slot4___N  rg_fruit=crop_GH1_NFT_slot4___rg_fruit  c_fruit_m=crop_GH1_NFT_slot4___c_fruit_m  c_fruit_g=crop_GH1_NFT_slot4___c_fruit_g  rg_leaf=crop_GH1_NFT_slot4___rg_leaf  c_leaf_m=crop_GH1_NFT_slot4___c_leaf_m  c_leaf_g=crop_GH1_NFT_slot4___c_leaf_g  rg_stem=crop_GH1_NFT_slot4___rg_stem  c_stem_m=crop_GH1_NFT_slot4___c_stem_m  c_stem_g=crop_GH1_NFT_slot4___c_stem_g  VelocityAbsortion=crop_GH1_NFT_slot4___VelocityAbsortion  T_max_v=crop_GH1_NFT_slot4___T_max_v  s_max_T=crop_GH1_NFT_slot4___s_max_T  s_min_T=crop_GH1_NFT_slot4___s_min_T  s_buforg_buf=crop_GH1_NFT_slot4___s_buforg_buf  T_sum_end=crop_GH1_NFT_slot4___T_sum_end  T_max_v24=crop_GH1_NFT_slot4___T_max_v24  T_min_v24=crop_GH1_NFT_slot4___T_min_v24  s_min_T24=crop_GH1_NFT_slot4___s_min_T24  s_max_T24=crop_GH1_NFT_slot4___s_max_T24  T_min_v=crop_GH1_NFT_slot4___T_min_v
      settings: SourceProductName=Horti Simulator
  Reorder signals : Subsystem
      settings: PortSchema="{\"entries\":[{\"content\":{\"sides\":[{\"content\":{\"connectorIds\":[\"In1\"]},\"type\":\"ConnectorPlacement.EquallySpacedRectSide\",\"uuid\":\"9bbb4059-7111-4f5f-880e-1e66f0dc329a\"},{\"content\":{\"connectorIds\":[\"Out1\",\"Out2\"],\"side\":\"RIGHT\"},\"type\":\"ConnectorPlacement.EquallySpacedRectSide\",\"uuid\":\"81ab22e8-385b-43c4-a26b-510ea5d440bf\"},{\"content\":{\"connectorIds\":[\"Out3\",\"Out4\"],\"side\":\"TOP\"},\"type\":\"ConnectorPlacement.EquallySpacedRectSide\",\"uuid\":\"0fc26091-ce19-4efa-b0aa-ccc08459932b\"},{\"content\":{\"connectorIds\":[\"In2\"],\"side\":\"BOTTOM\"},\"type\":\"ConnectorPlacement.EquallySpacedRectSide\",\"uuid\":\"583054f0-e45a-4f7d-ab46-2d52fcae7092\"}]},\"type\":\"ConnectorPlacement.EquallySpacedConnector\",\"uuid\":\"38c601a8-5a74-451d-8ace-3b63b0421924\"}],\"packageUris\":[\"http://schema.mathworks.com/mf0/Connector/R2020b\"],\"version\":\"1.0\"}"
  Tank Model : HORTISIM/Aquaculture/Models/Tank Model  S=tp_GH1_NFT___S  h_max=tp_GH1_NFT___h_max  wall_gain=tp_GH1_NFT___wall_gain  ThermalConductivityWall=tp_GH1_NFT___ThermalConductivityWall  Tsubwall=tp_GH1_NFT___Tsubwall  h=tp_GH1_NFT___h  X=tp_GH1_NFT___X  T=tp_GH1_NFT___T  Twall=tp_GH1_NFT___Twall  d_t=tp_GH1_NFT___d_t
      settings: SourceProductName=Horti Simulator
  Zero Element Flow2 : HORTISIM/Other  Functions/Zero Element Flow  SystemSampleTime=-1  VariantActivationTime=update diagram  Latency=0  AutoFrameSizeCalculation=off
      settings: SourceProductName=Horti Simulator
  subSelect Tank : HORTISIM/Other  Functions/subSelect  Tank  SystemSampleTime=-1  VariantActivationTime=update diagram  Latency=0  AutoFrameSizeCalculation=off
      settings: SourceProductName=Horti Simulator
  T : Outport
  CropInt : Outport  Port=2
  tag scope: GH1_NFT_C=global, TANK_GH1_NFT=global
  wires:
  f/1 -> Tank Model/1
  [IC] -> Tank Model/3
  Tank Model/1 -> subSelect Tank/1, T/1, [T]  "WT"
  [IC] -> Crop 1/1
  Control 1/1(CC) -> Crop 1/2
  Crop 1/1 -> [C1]  "Crop"
  Zero Element Flow2/1 -> Tank Model/2
  [C1] -> Control 1/1(Crop)
  IC/1 -> [IC]
  [IC] -> Crop 2/1
  Crop 2/1 -> [C2]  "Crop"
  [C2] -> Control 2/1(Crop)
  Control 2/1(CC) -> Crop 2/2
  [IC] -> Crop 3/1
  Crop 3/1 -> [C3]  "Crop"
  [C3] -> Control 3/1(Crop)
  Control 3/1(CC) -> Crop 3/2
  [IC] -> Crop 4/1
  Crop 4/1 -> [C4]  "Crop"
  [C4] -> Control 4/1(Crop)
  Control 4/1(CC) -> Crop 4/2
  [T] -> Reorder signals/2(WT)
  Reorder signals/3(fout) -> Tank Model/4
  Reorder signals/4(R) -> Tank Model/5
  Reorder signals/2(CropInt) -> CropInt/1
  Reorder signals/1(Subs) -> [Subs]
  [Subs] -> Bus Selector/1
  Bus Selector/1 -> Crop 1/3  "<Subs1>"
  [Subs] -> Bus Selector1/1
  Bus Selector1/1 -> Crop 3/3  "<Subs3>"
  [Subs] -> Bus Selector2/1
  Bus Selector2/1 -> Crop 4/3  "<Subs4>"
  [Subs] -> Bus Selector3/1
  Bus Selector3/1 -> Crop 2/3  "<Subs2>"
  [C1] -> Bus Creator/1
  [C4] -> Bus Creator/2  "Crop1"
  [C2] -> Bus Creator/3  "Crop2"
  [C3] -> Bus Creator/4  "Crop3"
  Bus Creator/1 -> Reorder signals/1(C1), [GH1_NFT_C]
  subSelect Tank/1 -> [TANK_GH1_NFT]

== system niof_model/GH1/Null Element ==
  Scalar2Bus Control Climate : HORTISIM/Other  Functions/Scalar2Bus  Control Climate  SystemSampleTime=-1  VariantActivationTime=update diagram  Latency=0  AutoFrameSizeCalculation=off
      settings: SourceProductName=Horti Simulator
  Zero Element Screen : HORTISIM/Other  Functions/Zero Element Screen  SystemSampleTime=-1  VariantActivationTime=update diagram  Latency=0  AutoFrameSizeCalculation=off
      settings: SourceProductName=Horti Simulator
  Zero Element Windows : HORTISIM/Other  Functions/Zero Element Windows  SystemSampleTime=-1  VariantActivationTime=update diagram  Latency=0  AutoFrameSizeCalculation=off
      link override Constant1: Value=1
      settings: SourceProductName=Horti Simulator
  CoCl : Outport
  wires:
  Scalar2Bus Control Climate/1 -> CoCl/1
  Zero Element Windows/1 -> Scalar2Bus Control Climate/1
  ? -> Scalar2Bus Control Climate/4
  ? -> Scalar2Bus Control Climate/3
  Zero Element Screen/1 -> Scalar2Bus Control Climate/2
